simulink model "Bicycle_model_constrained"  (R2020b)
settings: Solver=VariableStepAuto  StartTime=0.0  StopTime=10.0  RelTol=1e-3
model workspace (MAT data in the model file):
  Gravity = 9.81
  Mass = 285
  Weight_dist = 0.5
  Wheelbase = 1.35
libraries: simulink_extras x2
settings Model: OrderedModelArguments=off  Creator=yafta  LastModifiedBy=Matthew
settings ModelReferenceCC: ModelReferenceMinAlgLoopOccurrences=on

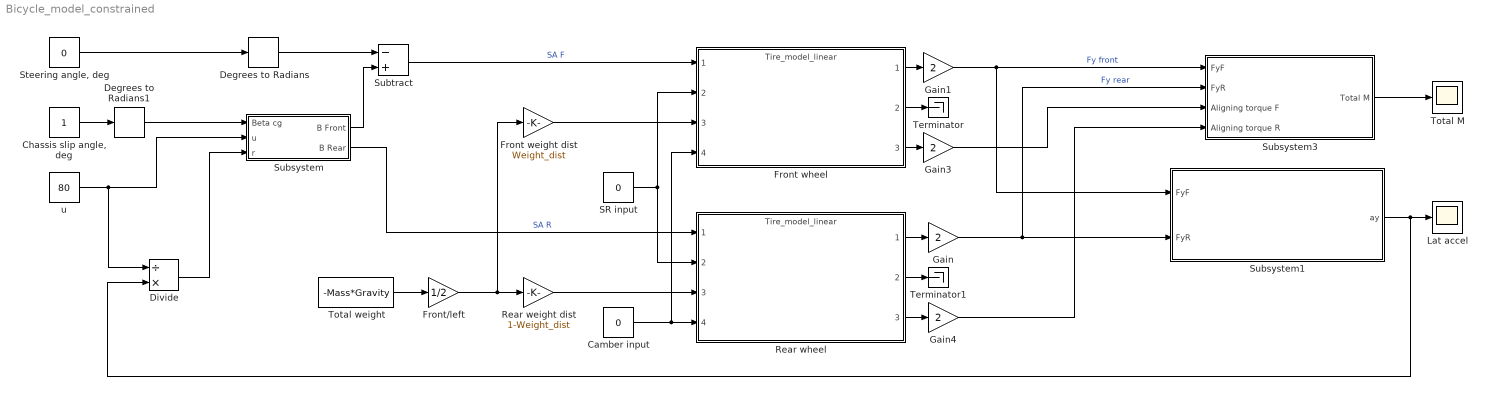
== system Bicycle_model_constrained ==
  Camber input : Constant  Value=0
  "Chassis slip angle, deg" : Constant
  Degrees to Radians : simulink_extras/Transformations/Degrees to Radians
  Degrees to Radians1 : simulink_extras/Transformations/Degrees to Radians
  Divide : Product  Inputs=/*
  Front weight dist : Gain  Gain=Weight_dist
  Front wheel : ModelReference  ModelNameDialog=Tire_model_linear.slx  UsingDefaultArgumentValue=0,0  SimulationMode=Normal  ModelReferenceVersion=2.10
  Front/left : Gain  Gain=1/2
  Gain{,1,3..4} (4 alike) : Gain  Gain=2
  Lat accel : Scope
  Rear weight dist : Gain  Gain=1-Weight_dist
  Rear wheel : ModelReference  ModelNameDialog=Tire_model_linear.slx  UsingDefaultArgumentValue=0,0  SimulationMode=Normal  ModelReferenceVersion=2.10
  SR input : Constant  Value=0
  "Steering angle, deg" : Constant  Value=0
  Subsystem : Subsystem
  Subsystem1 : Subsystem
  Subsystem3 : Subsystem
  Subtract : Sum  Inputs=-+
  Terminator : Terminator
  Terminator1 : Terminator
  Total M : Scope
  Total weight : Constant  Value=-Mass*Gravity
  u : Constant  Value=80
  wires:
  "Steering angle, deg"/1 -> Degrees to Radians/1
  Rear wheel/2 -> Terminator1/1
  Degrees to Radians1/1 -> Subsystem/1(Beta cg)
  Gain1/1 -> Subsystem3/1(FyF), Subsystem1/1(FyF)  "Fy front"
  Subsystem3/1(Total M) -> Total M/1
  Rear wheel/3 -> Gain4/1
  Divide/1 -> Subsystem/3(r)
  Subsystem1/1(ay) -> Divide/2, Lat accel/1
  Front wheel/2 -> Terminator/1
  "Chassis slip angle, deg"/1 -> Degrees to Radians1/1
  Total weight/1 -> Front/left/1
  Subsystem/2(B Rear) -> Rear wheel/1  "SA R"
  Rear wheel/1 -> Gain/1
  Gain4/1 -> Subsystem3/4(Aligning torque R)
  Front wheel/3 -> Gain3/1
  Gain/1 -> Subsystem3/2(FyR), Subsystem1/2(FyR)  "Fy rear"
  u/1 -> Divide/1, Subsystem/2(u)
  Subsystem/1(B Front) -> Subtract/2
  Degrees to Radians/1 -> Subtract/1
  Gain3/1 -> Subsystem3/3(Aligning torque F)
  Front weight dist/1 -> Front wheel/3
  Rear weight dist/1 -> Rear wheel/3
  Subtract/1 -> Front wheel/1  "SA F"
  SR input/1 -> Front wheel/2, Rear wheel/2
  Camber input/1 -> Rear wheel/4, Front wheel/4
  Front/left/1 -> Rear weight dist/1, Front weight dist/1
  Front wheel/1 -> Gain1/1

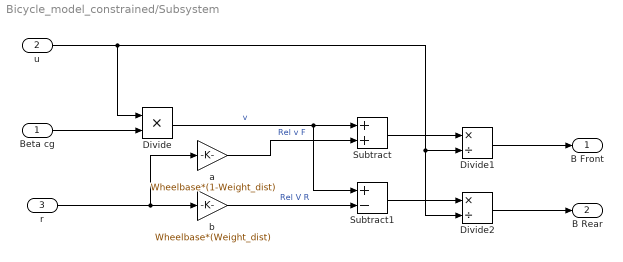
== system Bicycle_model_constrained/Subsystem ==
  Beta cg : Inport
  u : Inport  Port=2
  r : Inport  Port=3
  Divide : Product  Inputs=**
  Divide1 : Product  Inputs=*/
  Divide2 : Product  Inputs=*/
  Subtract : Sum
  Subtract1 : Sum  Inputs=+-
  a : Gain  Gain=Wheelbase*(1-Weight_dist)
  b : Gain  Gain=Wheelbase*(Weight_dist)
  B Front : Outport
  B Rear : Outport  Port=2
  wires:
  Divide/1 -> Subtract1/1, Subtract/1  "v"
  u/1 -> Divide/1, Divide2/2, Divide1/2
  r/1 -> a/1, b/1
  a/1 -> Subtract/2  "Rel v F"
  b/1 -> Subtract1/2  "Rel V R"
  Subtract/1 -> Divide1/1
  Subtract1/1 -> Divide2/1
  Beta cg/1 -> Divide/2
  Divide1/1 -> B Front/1
  Divide2/1 -> B Rear/1

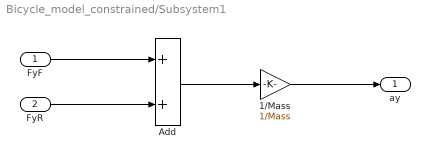
== system Bicycle_model_constrained/Subsystem1 ==
  FyF : Inport
  FyR : Inport  Port=2
  1/Mass : Gain  Gain=1/Mass
  Add : Sum
  ay : Outport
  wires:
  Add/1 -> 1/Mass/1
  1/Mass/1 -> ay/1
  FyR/1 -> Add/2
  FyF/1 -> Add/1

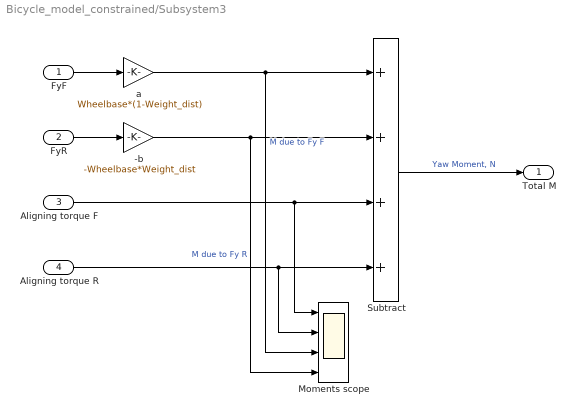
== system Bicycle_model_constrained/Subsystem3 ==
  FyF : Inport
  FyR : Inport  Port=2
  Aligning torque F : Inport  Port=3
  Aligning torque R : Inport  Port=4
  -b : Gain  Gain=-Wheelbase*Weight_dist
  Moments scope : Scope  NumInputPorts=4
  Subtract : Sum  Inputs=++++
  a : Gain  Gain=Wheelbase*(1-Weight_dist)
  Total M : Outport
  wires:
  -b/1 -> Moments scope/4, Subtract/2  "M due to Fy R"
  FyR/1 -> -b/1
  Aligning torque R/1 -> Subtract/4, Moments scope/2
  Subtract/1 -> Total M/1  "Yaw Moment, N"
  Aligning torque F/1 -> Moments scope/1, Subtract/3
  FyF/1 -> a/1
  a/1 -> Moments scope/3, Subtract/1  "M due to Fy F"
